simulink model "Vedant3112"  (R2018b)
settings: Solver=VariableStepAuto  StartTime=0.0  StopTime=10.0  RelTol=1e-3
settings Model: Creator=student  LastModifiedBy=student

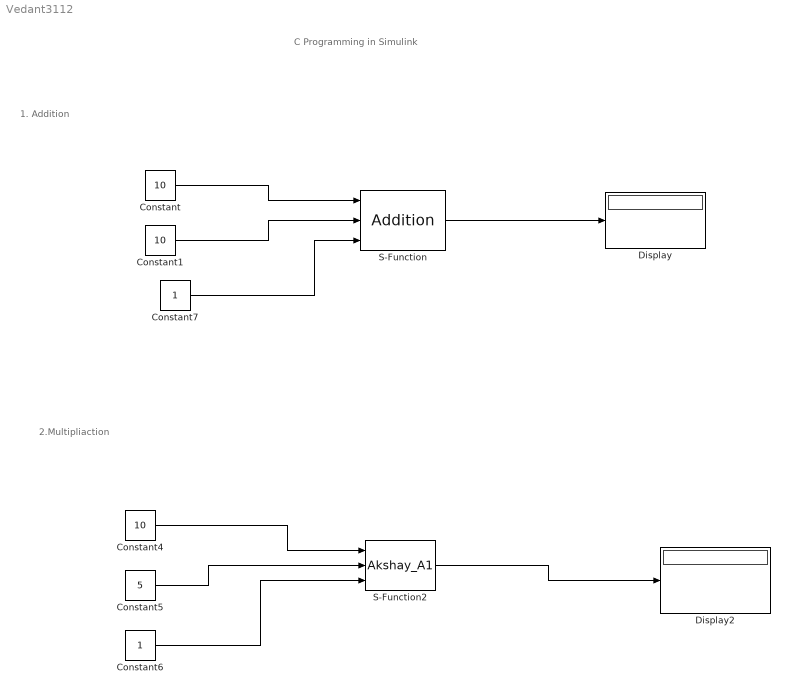
== system Vedant3112 ==
  note: 2.Multipliaction
  note: 1. Addition
  note: C Programming in Simulink
  Constant : Constant  Value=10
  Constant1 : Constant  Value=10
  Constant4 : Constant  Value=10
  Constant5 : Constant  Value=5
  Constant6 : Constant
  Constant7 : Constant
  Display : Display
  Display2 : Display
  S-Function : S-Function  FunctionName=Addition  SFunctionDeploymentMode=off  EnableBusSupport=off
  S-Function2 : S-Function  FunctionName=Akshay_A1  SFunctionDeploymentMode=off  EnableBusSupport=off
  wires:
  Constant/1 -> S-Function/1
  Constant1/1 -> S-Function/2
  S-Function/1 -> Display/1
  Constant6/1 -> S-Function2/3
  Constant5/1 -> S-Function2/2
  Constant4/1 -> S-Function2/1
  S-Function2/1 -> Display2/1
  Constant7/1 -> S-Function/3
